simulink model "mpc_tgt_calc"  (R2022b)
settings: Solver=FixedStepDiscrete  StartTime=0.0  StopTime=2600  FixedStep=0.1  RelTol=1e-3
undefined symbols (not defined in the file): accl, alpha, alpha2, ang, beta, cnt_delay_accl_ratio, cnt_delay_decel_ratio, delay_accl, delay_v, dist, dt, ff_duty_l, ff_duty_r, ideal_point, img_ang, img_dist, kanayama_point, pivot_state, sla_param, slip, slip_point, state, trj_diff, v, vx, vy, w
(part 2 of 2)

== system mpc_tgt_calc/slalom/Subsystem2 ==
  ego : Inport
  tgt : Inport  Port=2
  Add : Sum
  Add1 : Sum
  Bus Selector : BusSelector  OutputSignals=w,sla_param,sla_param.counter
  Bus Selector1 : BusSelector  OutputSignals=sla_param.counter,sla_param.limit_time_count
  Constant1 : Constant  Value=0
  Data Store Read : DataStoreRead  DataStoreName=time_step  IndexOptions=Index vector (dialog)  Indices=1  OutputSizes=1
  Data Store Read1 : DataStoreRead  DataStoreName=time_step  IndexOptions=Index vector (dialog)  Indices=1  OutputSizes=1
  Data Type Conversion : DataTypeConversion  OutDataTypeStr=single  SaturateOnIntegerOverflow=off  RndMeth=Floor
  Data Type Conversion1 : DataTypeConversion  OutDataTypeStr=single  SaturateOnIntegerOverflow=off  RndMeth=Floor
  Data Type Conversion2 : DataTypeConversion  OutDataTypeStr=single  SaturateOnIntegerOverflow=off  RndMeth=Floor
  Gain : Gain  Gain=dt
  Product : Product
  Relational Operator : RelationalOperator  OutDataTypeStr=boolean  RndMeth=Simplest  InputSameDT=off
  Subsystem : Subsystem
  Switch : Switch  Criteria=u2 > Threshold  SaturateOnIntegerOverflow=off  InputSameDT=off
  Terminator : Terminator
  next_w : Outport
  next_alpha : Outport  Port=2
  next_count : Outport  Port=3
  next_alpha2 : Outport  Port=4
  wires:
  Bus Selector/1 -> Add/1  "<w>"
  Subsystem/1(next_alpha) -> next_alpha/1, Gain/1
  Bus Selector/2 -> Subsystem/1(ego)  "<sla_param>"
  Bus Selector/3 -> Add1/1  "<counter>"
  Data Store Read1/1 -> Data Type Conversion2/1
  Add1/1 -> Data Type Conversion1/1
  Data Type Conversion/1 -> Add/2
  Data Type Conversion2/1 -> Add1/2
  Data Type Conversion1/1 -> next_count/1
  tgt/1 -> Terminator/1
  Bus Selector1/2 -> Relational Operator/2  "<limit_time_count>"
  Relational Operator/1 -> Switch/2
  ego/1 -> Bus Selector1/1, Bus Selector/1
  Bus Selector1/1 -> Relational Operator/1  "<counter>"
  Constant1/1 -> Switch/1
  Add/1 -> Switch/3
  Switch/1 -> next_w/1
  Data Store Read/1 -> Product/1
  Gain/1 -> Product/2
  Product/1 -> Data Type Conversion/1
  Subsystem/2(next_alpha2) -> next_alpha2/1

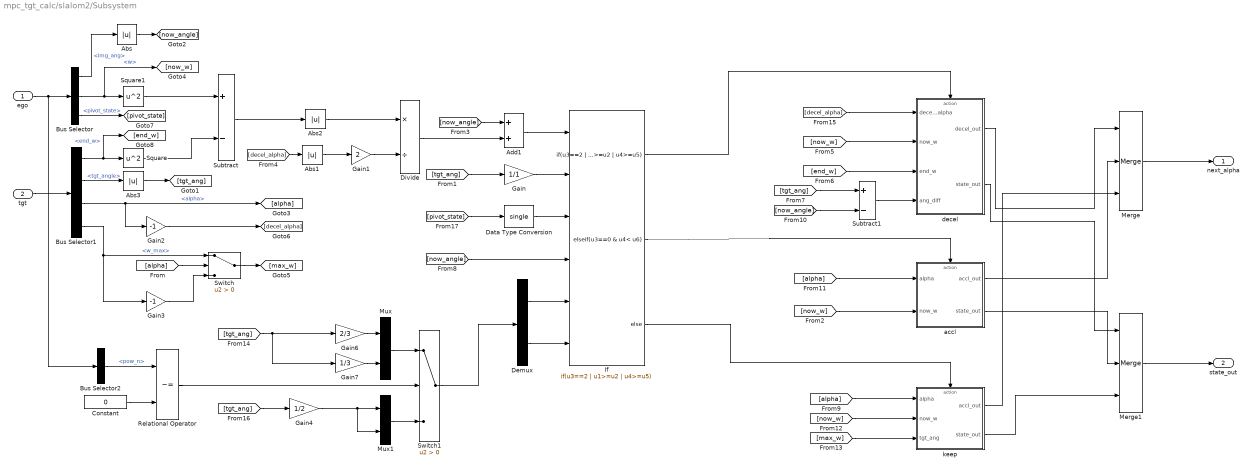
== system mpc_tgt_calc/slalom2/Subsystem ==
  ego : Inport
  tgt : Inport  Port=2
  Abs{,1..3} (4 alike) : Abs  SaturateOnIntegerOverflow=off
  Add1 : Sum
  Bus Selector : BusSelector  OutputSignals=img_ang,w,pivot_state
  Bus Selector1 : BusSelector  OutputSignals=end_w,tgt_angle,alpha,w_max
  Bus Selector2 : BusSelector  OutputSignals=sla_param.pow_n
  Constant : Constant  Value=0
  Data Type Conversion : DataTypeConversion  OutDataTypeStr=single  SaturateOnIntegerOverflow=off  RndMeth=Floor
  Demux : Demux  Outputs=2
  Divide : Product  Inputs=*/
  Gain : Gain  Gain=1/1
  Gain1 : Gain  Gain=2
  Gain2 : Gain  Gain=-1
  Gain3 : Gain  Gain=-1
  Gain4 : Gain  Gain=1/2
  Gain6 : Gain  Gain=2/3
  Gain7 : Gain  Gain=1/3
  If : If  NumInputs=6  IfExpression=u3==2 | u1>=u2 | u4>=u5  ElseIfExpressions=u3==0 & u4< u6
  Merge : Merge  Inputs=3
  Merge1 : Merge  Inputs=3
  Mux : Mux  Inputs=2
  Mux1 : Mux  Inputs=2
  Relational Operator : RelationalOperator  Operator=~=  OutDataTypeStr=boolean  RndMeth=Simplest  InputSameDT=off
  Square : Math  Operator=square
  Square1 : Math  Operator=square
  Subtract : Sum  Inputs=+-
  Subtract1 : Sum  Inputs=+-
  Switch : Switch  Criteria=u2 > Threshold  SaturateOnIntegerOverflow=off  InputSameDT=off
  Switch1 : Switch  Criteria=u2 > Threshold  SaturateOnIntegerOverflow=off  InputSameDT=off
  accl : Subsystem  TreatAsAtomicUnit=on
  decel : Subsystem  TreatAsAtomicUnit=on
  keep : Subsystem  TreatAsAtomicUnit=on
  next_alpha : Outport
  state_out : Outport  Port=2
  wires:
  ego/1 -> Bus Selector2/1, Bus Selector/1
  Subtract/1 -> Abs2/1
  Divide/1 -> Add1/2
  [now_angle] -> Add1/1
  Abs1/1 -> Gain1/1
  Abs2/1 -> Divide/1
  [decel_alpha] -> Abs1/1
  Gain1/1 -> Divide/2
  tgt/1 -> Bus Selector1/1
  Bus Selector1/1 -> [end_w], Square/1  "<end_w>"
  Square/1 -> Subtract/2
  Square1/1 -> Subtract/1
  Bus Selector/3 -> [pivot_state]  "<pivot_state>"
  Bus Selector/2 -> [now_w], Square1/1  "<w>"
  Bus Selector/1 -> Abs/1  "<img_ang>"
  Bus Selector1/2 -> Abs3/1  "<tgt_angle>"
  Bus Selector1/3 -> Gain2/1, [alpha]  "<alpha>"
  Gain2/1 -> [decel_alpha]
  Switch/1 -> [max_w]
  [alpha] -> Switch/2
  Bus Selector1/4 -> Gain3/1, Switch/1  "<w_max>"
  Gain3/1 -> Switch/3
  [pivot_state] -> Data Type Conversion/1
  Data Type Conversion/1 -> If/3
  Add1/1 -> If/1
  keep/2(state_out) -> Merge1/3
  decel/1(decel_out) -> Merge/1
  [max_w] -> keep/3(tgt_ang)
  accl/1(accl_out) -> Merge/2
  [now_w] -> keep/2(now_w)
  [decel_alpha] -> decel/1(decel_alpha)
  [now_w] -> decel/2(now_w)
  [now_angle] -> Subtract1/2
  [tgt_ang] -> Subtract1/1
  [now_w] -> accl/2(now_w)
  accl/2(state_out) -> Merge1/2
  If/2 -> accl/Action
  keep/1(accl_out) -> Merge/3
  [alpha] -> keep/1(alpha)
  If/3 -> keep/Action
  [end_w] -> decel/3(end_w)
  decel/2(state_out) -> Merge1/1
  Merge1/1 -> state_out/1
  Subtract1/1 -> decel/4(ang_diff)
  If/1 -> decel/Action
  Merge/1 -> next_alpha/1
  [alpha] -> accl/1(alpha)
  Abs/1 -> [now_angle]
  Abs3/1 -> [tgt_ang]
  Gain/1 -> If/2
  Demux/1 -> If/5
  [now_angle] -> If/4
  Demux/2 -> If/6
  [tgt_ang] -> Gain/1
  Gain7/1 -> Mux/2
  Gain6/1 -> Mux/1
  [tgt_ang] -> Gain6/1, Gain7/1
  Mux/1 -> Switch1/1
  Mux1/1 -> Switch1/3
  Gain4/1 -> Mux1/2, Mux1/1
  Switch1/1 -> Demux/1
  [tgt_ang] -> Gain4/1
  Bus Selector2/1 -> Relational Operator/1  "<pow_n>"
  Constant/1 -> Relational Operator/2
  Relational Operator/1 -> Switch1/2

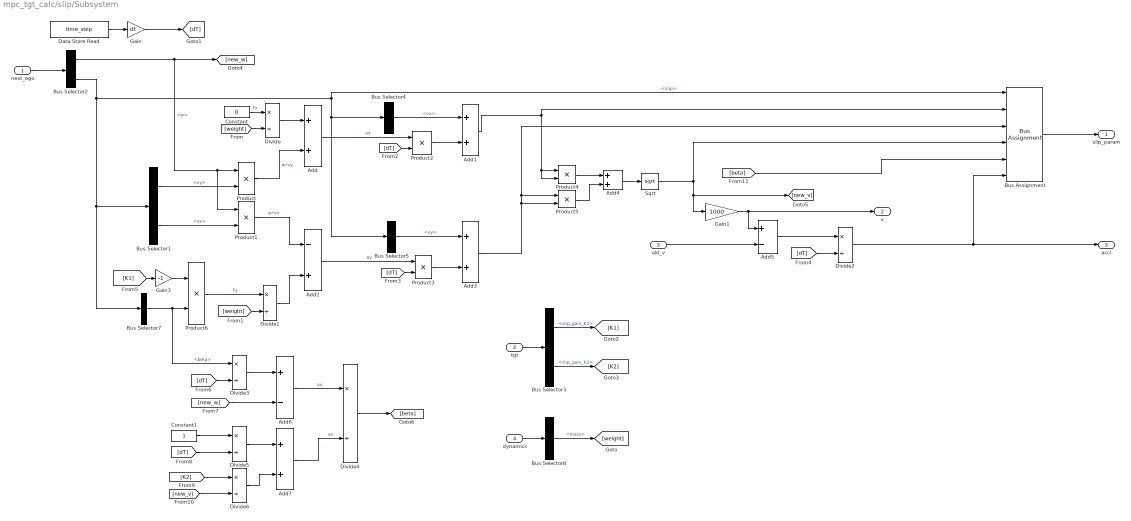
== system mpc_tgt_calc/slip/Subsystem ==
  next_ego : Inport
  tgt : Inport  Port=2
  old_v : Inport  Port=3
  dynamics : Inport  Port=4
  Add{,1,3..4,7} (5 alike) : Sum
  Add2 : Sum  Inputs=-+
  Add5 : Sum  Inputs=+-
  Add6 : Sum  Inputs=+-
  Bus Assignment : BusAssignment  AssignedSignals=vx,vy,v,beta,accl
  Bus Selector1 : BusSelector  OutputSignals=vy,vx
  Bus Selector2 : BusSelector  OutputSignals=w,slip
  Bus Selector3 : BusSelector  OutputSignals=slip_gain_K1,slip_gain_K2
  Bus Selector4 : BusSelector  OutputSignals=vx
  Bus Selector5 : BusSelector  OutputSignals=vy
  Bus Selector7 : BusSelector  OutputSignals=beta
  Bus Selector8 : BusSelector  OutputSignals=mass
  Constant : Constant  Value=0  OutDataTypeStr=single
  Constant1 : Constant  OutDataTypeStr=single
  Data Store Read : DataStoreRead  DataStoreName=time_step  IndexOptions=Index vector (dialog)  Indices=1  OutputSizes=1
  Divide{,1..6} (7 alike) : Product  Inputs=*/
  Gain : Gain  Gain=dt
  Gain1 : Gain  Gain=1000
  Gain3 : Gain  Gain=-1
  Product{,1..6} (7 alike) : Product
  Sqrt : Sqrt
  slip_param : Outport
  v : Outport  Port=2
  accl : Outport  Port=3
  wires:
  next_ego/1 -> Bus Selector2/1
  Bus Assignment/1 -> slip_param/1
  tgt/1 -> Bus Selector3/1
  Bus Selector2/1 -> [new_w], Product1/1, Product/1  "<w>"
  Bus Selector1/1 -> Product/2  "<vy>"
  Bus Selector1/2 -> Product1/2  "<vx>"
  Constant/1 -> Divide/1  "Fx"
  [weight] -> Divide/2
  [weight] -> Divide1/2
  Product/1 -> Add/2  "w*vy"
  Divide/1 -> Add/1
  Bus Selector4/1 -> Add1/1  "<vx>"
  Data Store Read/1 -> Gain/1
  Gain/1 -> [dT]
  Add/1 -> Product2/1  "ax"
  [dT] -> Product2/2
  Product2/1 -> Add1/2
  Add1/1 -> Product4/2, Product4/1, Bus Assignment/2
  Product3/1 -> Add3/2
  [dT] -> Product3/2
  Bus Selector2/2 -> Bus Selector7/1, Bus Selector1/1, Bus Assignment/1, Bus Selector4/1, Bus Selector5/1  "<slip>"
  Add3/1 -> Product5/1, Bus Assignment/3, Product5/2
  Add2/1 -> Product3/1  "ay"
  Bus Selector5/1 -> Add3/1  "<vy>"
  Product1/1 -> Add2/1  "w*vx"
  Product5/1 -> Add4/2
  Sqrt/1 -> [new_v], Gain1/1, Bus Assignment/4
  Add4/1 -> Sqrt/1
  Product4/1 -> Add4/1
  Gain1/1 -> Add5/1, v/1
  Divide1/1 -> Add2/2
  old_v/1 -> Add5/2
  Add5/1 -> Divide2/1
  [dT] -> Divide2/2
  Divide2/1 -> Bus Assignment/6, accl/1
  Bus Selector3/1 -> [K1]  "<slip_gain_K1>"
  Bus Selector3/2 -> [K2]  "<slip_gain_K2>"
  Gain3/1 -> Product6/1
  [K1] -> Gain3/1
  Bus Selector7/1 -> Divide3/1, Product6/2  "<beta>"
  Product6/1 -> Divide1/1  "Fy"
  [dT] -> Divide3/2
  [new_w] -> Add6/2
  Divide3/1 -> Add6/1
  Add6/1 -> Divide4/1  "ax"
  [dT] -> Divide5/2
  Constant1/1 -> Divide5/1
  Divide5/1 -> Add7/1
  Divide6/1 -> Add7/2
  Add7/1 -> Divide4/2  "ax"
  [K2] -> Divide6/1
  [new_v] -> Divide6/2
  Divide4/1 -> [beta]
  [beta] -> Bus Assignment/5
  dynamics/1 -> Bus Selector8/1
  Bus Selector8/1 -> [weight]  "<mass>"

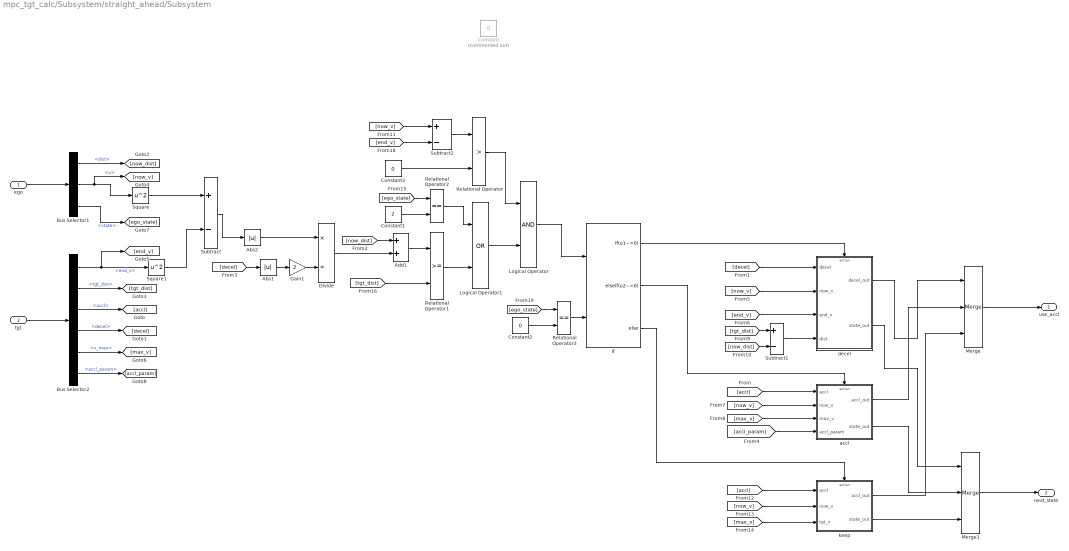
== system mpc_tgt_calc/Subsystem/straight_ahead/Subsystem ==
  ego : Inport
  tgt : Inport  Port=2
  Abs1 : Abs  SaturateOnIntegerOverflow=off
  Abs2 : Abs  SaturateOnIntegerOverflow=off
  Add1 : Sum
  Bus Selector1 : BusSelector  OutputSignals=dist,v,state
  Bus Selector2 : BusSelector  OutputSignals=end_v,tgt_dist,accl,decel,v_max,accl_param
  Constant : Constant  Commented=on  Value=0
  Constant1 : Constant  Value=2
  Constant2 : Constant  Value=0
  Constant3 : Constant  Value=0
  Divide : Product  Inputs=*/
  Gain1 : Gain  Gain=2
  If : If  NumInputs=2  IfExpression=u1~=0  ElseIfExpressions=u2~=0
  Logical Operator : Logic  AllPortsSameDT=off  OutDataTypeStr=boolean
  Logical Operator1 : Logic  Operator=OR  AllPortsSameDT=off  OutDataTypeStr=boolean
  Merge : Merge  Inputs=3
  Merge1 : Merge  Inputs=3
  Relational Operator : RelationalOperator  Operator=>  OutDataTypeStr=boolean  RndMeth=Simplest  InputSameDT=off
  Relational Operator1 : RelationalOperator  OutDataTypeStr=boolean  RndMeth=Simplest  InputSameDT=off
  Relational Operator2 : RelationalOperator  Operator===  OutDataTypeStr=boolean  RndMeth=Simplest  InputSameDT=off
  Relational Operator3 : RelationalOperator  Operator===  OutDataTypeStr=boolean  RndMeth=Simplest  InputSameDT=off
  Square : Math  Operator=square
  Square1 : Math  Operator=square
  Subtract : Sum  Inputs=+-
  Subtract1 : Sum  Inputs=+-
  Subtract2 : Sum  Inputs=+-
  accl : Subsystem  TreatAsAtomicUnit=on
  decel : Subsystem  TreatAsAtomicUnit=on
  keep : Subsystem  TreatAsAtomicUnit=on
  use_accl : Outport
  next_state : Outport  Port=2
  wires:
  Add1/1 -> Relational Operator1/1
  Gain1/1 -> Divide/2
  tgt/1 -> Bus Selector2/1
  [accl] -> accl/1(accl)
  [decel] -> decel/1(decel)
  Square/1 -> Subtract/1
  Divide/1 -> Add1/2
  Bus Selector2/1 -> [end_v], Square1/1  "<end_v>"
  ego/1 -> Bus Selector1/1
  Bus Selector1/2 -> Square/1, [now_v]  "<v>"
  Bus Selector2/3 -> [accl]  "<accl>"
  Bus Selector2/4 -> [decel]  "<decel>"
  Bus Selector1/1 -> [now_dist]  "<dist>"
  [now_dist] -> Add1/1
  [decel] -> Abs1/1
  Abs1/1 -> Gain1/1
  Subtract/1 -> Abs2/1
  Bus Selector2/2 -> [tgt_dist]  "<tgt_dist>"
  [now_v] -> decel/2(now_v)
  [end_v] -> decel/3(end_v)
  [now_v] -> accl/2(now_v)
  Bus Selector2/5 -> [max_v]  "<v_max>"
  Bus Selector1/3 -> [ego_state]  "<state>"
  Merge/1 -> use_accl/1
  [tgt_dist] -> Subtract1/1
  [now_dist] -> Subtract1/2
  Subtract1/1 -> decel/4(dist)
  [max_v] -> accl/3(max_v)
  If/3 -> keep/Action
  Merge1/1 -> next_state/1
  [accl] -> keep/1(accl)
  [now_v] -> keep/2(now_v)
  [max_v] -> keep/3(tgt_v)
  If/1 -> decel/Action
  If/2 -> accl/Action
  keep/1(accl_out) -> Merge/3
  decel/1(decel_out) -> Merge/1
  decel/2(state_out) -> Merge1/1
  keep/2(state_out) -> Merge1/3
  accl/1(accl_out) -> Merge/2
  accl/2(state_out) -> Merge1/2
  Bus Selector2/6 -> [accl_param]  "<accl_param>"
  [accl_param] -> accl/4(accl_param)
  [now_v] -> Subtract2/1
  [end_v] -> Subtract2/2
  Subtract2/1 -> Relational Operator/1
  Square1/1 -> Subtract/2
  Constant3/1 -> Relational Operator/2
  Relational Operator/1 -> Logical Operator/1
  [tgt_dist] -> Relational Operator1/2
  Relational Operator1/1 -> Logical Operator1/2
  [ego_state] -> Relational Operator2/1
  Constant1/1 -> Relational Operator2/2
  Relational Operator2/1 -> Logical Operator1/1
  Logical Operator1/1 -> Logical Operator/2
  Logical Operator/1 -> If/1
  [ego_state] -> Relational Operator3/1
  Relational Operator3/1 -> If/2
  Constant2/1 -> Relational Operator3/2
  Abs2/1 -> Divide/1

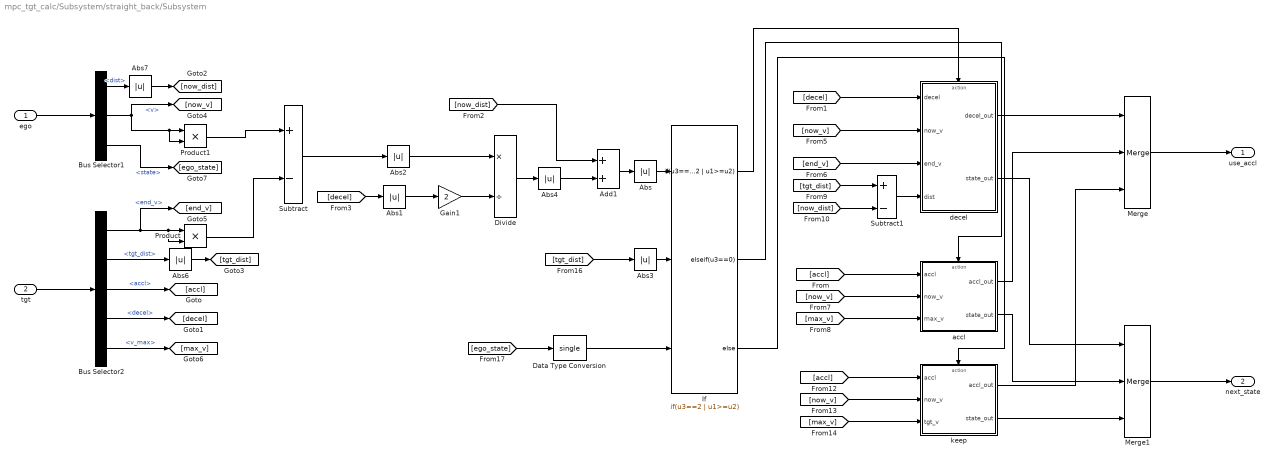
== system mpc_tgt_calc/Subsystem/straight_back/Subsystem ==
  ego : Inport
  tgt : Inport  Port=2
  Abs{,1..4,6..7} (7 alike) : Abs  SaturateOnIntegerOverflow=off
  Add1 : Sum
  Bus Selector1 : BusSelector  OutputSignals=dist,v,state
  Bus Selector2 : BusSelector  OutputSignals=end_v,tgt_dist,accl,decel,v_max
  Data Type Conversion : DataTypeConversion  OutDataTypeStr=single  SaturateOnIntegerOverflow=off  RndMeth=Floor
  Divide : Product  Inputs=*/
  Gain1 : Gain  Gain=2
  If : If  NumInputs=3  IfExpression=u3==2 | u1>=u2  ElseIfExpressions=u3==0
  Merge : Merge  Inputs=3
  Merge1 : Merge  Inputs=3
  Product : Product
  Product1 : Product
  Subtract : Sum  Inputs=+-
  Subtract1 : Sum  Inputs=+-
  accl : Subsystem  TreatAsAtomicUnit=on
  decel : Subsystem  TreatAsAtomicUnit=on
  keep : Subsystem  TreatAsAtomicUnit=on
  use_accl : Outport
  next_state : Outport  Port=2
  wires:
  Add1/1 -> Abs/1
  Gain1/1 -> Divide/2
  Product/1 -> Subtract/2
  Subtract/1 -> Abs2/1
  tgt/1 -> Bus Selector2/1
  [accl] -> accl/1(accl)
  [decel] -> decel/1(decel)
  Product1/1 -> Subtract/1
  Divide/1 -> Abs4/1
  Bus Selector2/1 -> Product/2, Product/1, [end_v]  "<end_v>"
  ego/1 -> Bus Selector1/1
  Bus Selector1/2 -> Product1/2, Product1/1, [now_v]  "<v>"
  Bus Selector2/3 -> [accl]  "<accl>"
  Bus Selector2/4 -> [decel]  "<decel>"
  Bus Selector1/1 -> Abs7/1  "<dist>"
  [decel] -> Abs1/1
  Abs1/1 -> Gain1/1
  Abs2/1 -> Divide/1
  Bus Selector2/2 -> Abs6/1  "<tgt_dist>"
  [now_v] -> decel/2(now_v)
  [end_v] -> decel/3(end_v)
  [now_v] -> accl/2(now_v)
  Bus Selector2/5 -> [max_v]  "<v_max>"
  Bus Selector1/3 -> [ego_state]  "<state>"
  Merge/1 -> use_accl/1
  [tgt_dist] -> Subtract1/1
  [now_dist] -> Subtract1/2
  Subtract1/1 -> decel/4(dist)
  [max_v] -> accl/3(max_v)
  If/3 -> keep/Action
  Merge1/1 -> next_state/1
  [accl] -> keep/1(accl)
  [now_v] -> keep/2(now_v)
  [max_v] -> keep/3(tgt_v)
  If/1 -> decel/Action
  If/2 -> accl/Action
  [tgt_dist] -> Abs3/1
  [ego_state] -> Data Type Conversion/1
  Data Type Conversion/1 -> If/3
  keep/1(accl_out) -> Merge/3
  decel/1(decel_out) -> Merge/1
  decel/2(state_out) -> Merge1/1
  keep/2(state_out) -> Merge1/3
  accl/1(accl_out) -> Merge/2
  accl/2(state_out) -> Merge1/2
  Abs/1 -> If/1
  Abs3/1 -> If/2
  Abs4/1 -> Add1/2
  [now_dist] -> Add1/1
  Abs6/1 -> [tgt_dist]
  Abs7/1 -> [now_dist]

== system mpc_tgt_calc/calc_FF/Subsystem/If Action Subsystem ==
  front_volt : Inport
  next_ego : Inport  Port=2
  Action Port : ActionPort  ActionPortLabel=if((u2==0 | u2==3 ) & (u1==0))
  Bus Selector : BusSelector  OutputSignals=ff_duty_low_v_th,ff_duty_low_th
  Bus Selector1 : BusSelector  OutputSignals=v
  Max : MinMax  Function=max  Inputs=2
  Mux : Mux  Inputs=2
  Relational Operator : RelationalOperator  Operator=>  OutDataTypeStr=boolean  RndMeth=Simplest  InputSameDT=off
  Scope : Scope  NumInputPorts=4
  Switch : Switch  Criteria=u2 > Threshold  SaturateOnIntegerOverflow=off  InputSameDT=off
  Out1 : Outport
  wires:
  next_ego/1 -> Bus Selector/1, Bus Selector1/1
  Bus Selector1/1 -> Mux/1, Relational Operator/1  "<v>"
  Bus Selector/1 -> Mux/2, Relational Operator/2  "<ff_duty_low_v_th>"
  Relational Operator/1 -> Scope/3, Switch/2
  front_volt/1 -> Max/1, Switch/1
  Bus Selector/2 -> Max/2  "<ff_duty_low_th>"
  Switch/1 -> Scope/1, Out1/1
  Max/1 -> Scope/2, Switch/3
  Mux/1 -> Scope/4

== system mpc_tgt_calc/calc_FF/Subsystem/If Action Subsystem1 ==
  front_volt : Inport
  Action Port : ActionPort  ActionPortLabel=else
  Out1 : Outport
  wires:
  front_volt/1 -> Out1/1

== system mpc_tgt_calc/pivot/Subsystem/accl ==
  alpha : Inport
  now_w : Inport  Port=2
  max_w : Inport  Port=3
  Action Port : ActionPort  ActionPortLabel=elseif(u3==0 )
  Abs : Abs  SaturateOnIntegerOverflow=off
  Abs1 : Abs  SaturateOnIntegerOverflow=off
  Constant : Constant  Value=0
  Constant1 : Constant  Value=0  OutDataTypeStr=int32
  Constant2 : Constant  OutDataTypeStr=int32
  Constant3 : Constant  OutDataTypeStr=single
  Constant4 : Constant  Value=2.5  OutDataTypeStr=single
  Data Type Conversion : DataTypeConversion  OutDataTypeStr=single  SaturateOnIntegerOverflow=off  RndMeth=Floor
  Divide : Product  Inputs=*/
  Manual Switch : ManualSwitch
  Product1 : Product
  Relational Operator : RelationalOperator  Operator=<  OutDataTypeStr=boolean  RndMeth=Simplest  InputSameDT=off
  Square : Math  Operator=pow
  Subtract : Sum  Inputs=+-
  Switch : Switch  Criteria=u2 > Threshold  SaturateOnIntegerOverflow=off  InputSameDT=off
  Switch1 : Switch  Criteria=u2 > Threshold  SaturateOnIntegerOverflow=off  InputSameDT=off
  accl_out : Outport
  state_out : Outport  Port=2
  wires:
  Switch/1 -> Data Type Conversion/1
  Relational Operator/1 -> Switch1/2, Switch/2
  max_w/1 -> Divide/2, Abs1/1
  Constant/1 -> Switch/3
  alpha/1 -> [alpha], Manual Switch/1, Product1/1
  Constant1/1 -> Switch1/1
  Constant2/1 -> Switch1/3
  Constant3/1 -> Subtract/1
  Divide/1 -> Square/1
  Square/1 -> Subtract/2
  Subtract/1 -> Product1/2
  Constant4/1 -> Square/2
  Product1/1 -> Manual Switch/2
  Manual Switch/1 -> Switch/1
  now_w/1 -> Abs/1, Divide/1
  Switch1/1 -> state_out/1
  Data Type Conversion/1 -> accl_out/1
  Abs/1 -> Relational Operator/1
  Abs1/1 -> Relational Operator/2

== system mpc_tgt_calc/pivot/Subsystem/decel ==
  decel_alpha : Inport
  now_w : Inport  Port=2
  end_w : Inport  Port=3
  ang : Inport  Port=4
  Action Port : ActionPort  ActionPortLabel=if(u3==2 | u1>=u2)
  Abs : Abs  SaturateOnIntegerOverflow=off
  Abs1 : Abs  SaturateOnIntegerOverflow=off
  Abs2 : Abs  SaturateOnIntegerOverflow=off
  Constant : Constant  Value=0  OutDataTypeStr=single
  Constant1 : Constant  Value=0.01*2*pi/360
  Constant2 : Constant  Value=2  OutDataTypeStr=int32
  Data Type Conversion : DataTypeConversion  OutDataTypeStr=single  SaturateOnIntegerOverflow=off  RndMeth=Floor
  Divide : Product  Inputs=*/
  Gain : Gain  Gain=2
  Gain1 : Gain  Gain=-1
  Manual Switch : ManualSwitch  CurrentSetting=0
  Min : MinMax  Function=max  Inputs=2
  Relational Operator : RelationalOperator  Operator=>  OutDataTypeStr=boolean  RndMeth=Simplest  InputSameDT=off
  Relational Operator1 : RelationalOperator  Operator=<  OutDataTypeStr=boolean  RndMeth=Simplest  InputSameDT=off
  Relational Operator2 : RelationalOperator  Operator=<  OutDataTypeStr=boolean  RndMeth=Simplest  InputSameDT=off
  Square : Math  Operator=square
  Square1 : Math  Operator=square
  Subtract : Sum  Inputs=+-
  Switch{,1..3} (4 alike) : Switch  Criteria=u2 > Threshold  SaturateOnIntegerOverflow=off  InputSameDT=off
  decel_out : Outport
  state_out : Outport  Port=2
  wires:
  Square1/1 -> Subtract/2
  Constant1/1 -> Min/1
  Min/1 -> Gain/1
  Subtract/1 -> Divide/1
  Constant/1 -> Switch/3
  Gain/1 -> Divide/2
  Divide/1 -> Abs/1
  ang/1 -> Min/2
  Square/1 -> Subtract/1
  Constant2/1 -> state_out/1
  end_w/1 -> Relational Operator/2, Relational Operator1/2, Square1/1
  now_w/1 -> Relational Operator/1, Relational Operator1/1, Square/1
  [decel_alpha] -> Switch2/2
  Relational Operator/1 -> Switch2/3
  Relational Operator1/1 -> Switch2/1
  Switch1/1 -> Manual Switch/2
  Abs/1 -> Data Type Conversion/1
  Gain1/1 -> Switch1/3
  Switch2/1 -> Switch/2
  Switch/1 -> decel_out/1
  Data Type Conversion/1 -> Gain1/1, Switch1/1
  Manual Switch/1 -> Switch/1, Abs1/1
  decel_alpha/1 -> [decel_alpha], Switch1/2, Switch3/1, Abs2/1, Manual Switch/1
  Abs2/1 -> Relational Operator2/1
  Relational Operator2/1 -> Switch3/2
  Abs1/1 -> Relational Operator2/2

== system mpc_tgt_calc/pivot/Subsystem/keep ==
  alpha : Inport
  now_w : Inport  Port=2
  tgt_ang : Inport  Port=3
  Action Port : ActionPort  ActionPortLabel=else
  Constant : Constant  Value=0
  Constant2 : Constant  OutDataTypeStr=int32
  Data Type Conversion : DataTypeConversion  OutDataTypeStr=single  SaturateOnIntegerOverflow=off  RndMeth=Floor
  Terminator : Terminator
  Terminator1 : Terminator
  Terminator2 : Terminator
  accl_out : Outport
  state_out : Outport  Port=2
  wires:
  Constant2/1 -> state_out/1
  Constant/1 -> Data Type Conversion/1
  Data Type Conversion/1 -> accl_out/1
  alpha/1 -> Terminator/1
  now_w/1 -> Terminator1/1
  tgt_ang/1 -> Terminator2/1

== system mpc_tgt_calc/slalom/Subsystem2/Subsystem ==
  ego : Inport
  Add : Sum
  Add1 : Sum
  Bus Selector : BusSelector  OutputSignals=state,base_alpha,counter,limit_time_count
  Constant : Constant  Value=0  OutDataTypeStr=single
  Data Store Read1 : DataStoreRead  DataStoreName=time_step  IndexOptions=Index vector (dialog)  Indices=1  OutputSizes=1
  Data Store Read2 : DataStoreRead  DataStoreName=time_step2  IndexOptions=Index vector (dialog)  Indices=1  OutputSizes=1
  If : If  IfExpression=u1 ~= 0
  If Action Subsystem : Subsystem  TreatAsAtomicUnit=on
  If Action Subsystem1 : Subsystem  TreatAsAtomicUnit=on
  If Action Subsystem2 : Subsystem  TreatAsAtomicUnit=on
  If Action Subsystem3 : Subsystem  TreatAsAtomicUnit=on
  If2 : If  IfExpression=u1 ~= 0
  Merge : Merge
  Merge1 : Merge
  Product : Product
  Product1 : Product
  Relational Operator : RelationalOperator  Operator=>  OutDataTypeStr=boolean  RndMeth=Simplest  InputSameDT=off
  Relational Operator1 : RelationalOperator  Operator=>  OutDataTypeStr=boolean  RndMeth=Simplest  InputSameDT=off
  Switch : Switch  Criteria=u2 ~= 0  SaturateOnIntegerOverflow=off  InputSameDT=off
  Switch3 : Switch  Criteria=u2 ~= 0  SaturateOnIntegerOverflow=off  InputSameDT=off
  next_alpha : Outport
  next_alpha2 : Outport  Port=2
  wires:
  ego/1 -> If Action Subsystem3/1(ego), If Action Subsystem1/1(ego), Bus Selector/1
  Bus Selector/1 -> Switch3/2, Switch/2  "<state>"
  Switch/1 -> next_alpha/1
  Constant/1 -> Switch3/1, Switch/1
  Bus Selector/2 -> Product1/1, Product/1  "<base_alpha>"
  Product/1 -> Switch/3
  Merge/1 -> Product/2
  Relational Operator/1 -> If/1
  Bus Selector/4 -> Relational Operator1/2, Relational Operator/2  "<limit_time_count>"
  Data Store Read1/1 -> Add/1
  Bus Selector/3 -> Add1/2, Add/2  "<counter>"
  Add/1 -> Relational Operator/1
  Product1/1 -> Switch3/3
  Switch3/1 -> next_alpha2/1
  Data Store Read2/1 -> Add1/1
  Add1/1 -> Relational Operator1/1
  If/1 -> If Action Subsystem/Action
  Relational Operator1/1 -> If2/1
  If/2 -> If Action Subsystem1/Action
  If Action Subsystem/1(Out1) -> Merge/1
  If Action Subsystem1/1(neipier) -> Merge/2
  If Action Subsystem2/1(Out1) -> Merge1/1
  If2/1 -> If Action Subsystem2/Action
  If Action Subsystem3/1(neipier) -> Merge1/2
  If2/2 -> If Action Subsystem3/Action
  Merge1/1 -> Product1/2

== system mpc_tgt_calc/slalom2/Subsystem/accl ==
  alpha : Inport
  now_w : Inport  Port=2
  Action Port : ActionPort  ActionPortLabel=elseif(u3==0 & u4< u6)
  Constant1 : Constant  Value=0  OutDataTypeStr=int32
  Data Type Conversion : DataTypeConversion  OutDataTypeStr=single  SaturateOnIntegerOverflow=off  RndMeth=Floor
  Terminator : Terminator
  accl_out : Outport
  state_out : Outport  Port=2
  wires:
  alpha/1 -> Data Type Conversion/1
  Constant1/1 -> state_out/1
  Data Type Conversion/1 -> accl_out/1
  now_w/1 -> Terminator/1

== system mpc_tgt_calc/slalom2/Subsystem/decel ==
  decel_alpha : Inport
  now_w : Inport  Port=2
  end_w : Inport  Port=3
  ang_diff : Inport  Port=4
  Action Port : ActionPort  ActionPortLabel=if(u3==2 | u1>=u2 | u4>=u5)
  Abs : Abs  SaturateOnIntegerOverflow=off
  Constant : Constant  Value=0  OutDataTypeStr=single
  Constant1 : Constant  Value=0.1*pi/180
  Constant2 : Constant  Value=2  OutDataTypeStr=int32
  Constant3 : Constant  Commented=on  Value=0.75
  Data Type Conversion : DataTypeConversion  OutDataTypeStr=single  SaturateOnIntegerOverflow=off  RndMeth=Floor
  Divide : Product  Inputs=*/
  From1 : From  Commented=on  GotoTag=ang_diff_abs
  Gain : Gain  Gain=2
  Gain1 : Gain  Gain=-1
  Min : MinMax  Function=max  Inputs=2
  Relational Operator : RelationalOperator  Operator=>  OutDataTypeStr=boolean  RndMeth=Simplest  InputSameDT=off
  Relational Operator1 : RelationalOperator  Operator=<  OutDataTypeStr=boolean  RndMeth=Simplest  InputSameDT=off
  Relational Operator2 : RelationalOperator  Commented=on  Operator=>  OutDataTypeStr=boolean  RndMeth=Simplest  InputSameDT=off
  Square : Math  Operator=square
  Square1 : Math  Operator=square
  Subtract : Sum  Inputs=+-
  Switch : Switch  Criteria=u2 > Threshold  SaturateOnIntegerOverflow=off  InputSameDT=off
  Switch1 : Switch  Criteria=u2 > Threshold  SaturateOnIntegerOverflow=off  InputSameDT=off
  Switch2 : Switch  Criteria=u2 > Threshold  SaturateOnIntegerOverflow=off  InputSameDT=off
  Switch3 : Switch  Commented=on  Criteria=u2 > Threshold  SaturateOnIntegerOverflow=off  InputSameDT=off
  decel_out : Outport
  state_out : Outport  Port=2
  wires:
  Square1/1 -> Subtract/2
  ang_diff/1 -> Min/1
  Min/1 -> Gain/1
  Subtract/1 -> Divide/1
  Constant/1 -> Switch/3
  Gain/1 -> Divide/2
  Divide/1 -> Abs/1
  Square/1 -> Subtract/1
  Constant2/1 -> state_out/1
  decel_alpha/1 -> [decel_alpha], Switch1/2, Switch3/1
  end_w/1 -> Relational Operator/2, Relational Operator1/2, Square1/1
  now_w/1 -> Relational Operator/1, Relational Operator1/1, Square/1
  [decel_alpha] -> Switch2/2
  Relational Operator/1 -> Switch2/3
  Relational Operator1/1 -> Switch2/1
  Switch1/1 -> Switch/1
  Abs/1 -> Data Type Conversion/1
  Gain1/1 -> Switch1/3
  Switch2/1 -> Switch/2
  Switch/1 -> decel_out/1
  Data Type Conversion/1 -> Gain1/1, Switch1/1
  From1/1 -> Relational Operator2/1
  Constant3/1 -> Relational Operator2/2
  Relational Operator2/1 -> Switch3/2
  Constant1/1 -> Min/2

== system mpc_tgt_calc/slalom2/Subsystem/keep ==
  alpha : Inport
  now_w : Inport  Port=2
  tgt_ang : Inport  Port=3
  Action Port : ActionPort  ActionPortLabel=else
  Constant : Constant  Value=0
  Constant2 : Constant  OutDataTypeStr=int32
  Data Type Conversion : DataTypeConversion  OutDataTypeStr=single  SaturateOnIntegerOverflow=off  RndMeth=Floor
  Terminator : Terminator
  Terminator1 : Terminator
  Terminator2 : Terminator
  accl_out : Outport
  state_out : Outport  Port=2
  wires:
  Constant2/1 -> state_out/1
  Constant/1 -> Data Type Conversion/1
  Data Type Conversion/1 -> accl_out/1
  alpha/1 -> Terminator/1
  now_w/1 -> Terminator1/1
  tgt_ang/1 -> Terminator2/1

== system mpc_tgt_calc/Subsystem/straight_ahead/Subsystem/accl ==
  accl : Inport
  now_v : Inport  Port=2
  max_v : Inport  Port=3
  accl_param : Inport  Port=4
  Action Port : ActionPort  ActionPortLabel=elseif(u2~=0 )
  Bus Selector : BusSelector  OutputSignals=limit,n
  Constant : Constant  Value=0
  Constant1 : Constant  Value=0  OutDataTypeStr=int32
  Constant2 : Constant  OutDataTypeStr=int32
  Constant3 : Constant  OutDataTypeStr=single
  Data Type Conversion : DataTypeConversion  OutDataTypeStr=single  SaturateOnIntegerOverflow=off  RndMeth=Floor
  Divide : Product  Inputs=*/
  Product1 : Product
  Relational Operator : RelationalOperator  Operator=<  OutDataTypeStr=boolean  RndMeth=Simplest  InputSameDT=off
  Relational Operator1 : RelationalOperator  Operator=>  OutDataTypeStr=boolean  RndMeth=Simplest  InputSameDT=off
  Square : Math  Operator=pow
  Subtract : Sum  Inputs=+-
  Switch : Switch  Criteria=u2 > Threshold  SaturateOnIntegerOverflow=off  InputSameDT=off
  Switch1 : Switch  Criteria=u2 > Threshold  SaturateOnIntegerOverflow=off  InputSameDT=off
  Switch2 : Switch  Criteria=u2 > Threshold  SaturateOnIntegerOverflow=off  InputSameDT=off
  accl_out : Outport
  state_out : Outport  Port=2
  wires:
  Switch/1 -> Data Type Conversion/1
  now_v/1 -> Relational Operator1/1, Relational Operator/1, Divide/1
  Relational Operator/1 -> Switch/2, Switch1/2
  max_v/1 -> Relational Operator/2, Divide/2
  Constant/1 -> Switch/3
  Data Type Conversion/1 -> accl_out/1
  accl/1 -> Switch2/3, Product1/1
  Switch1/1 -> state_out/1
  Constant1/1 -> Switch1/1
  Constant2/1 -> Switch1/3
  Constant3/1 -> Subtract/1
  Divide/1 -> Square/1
  Square/1 -> Subtract/2
  Subtract/1 -> Product1/2
  [n] -> Square/2
  Switch2/1 -> Switch/1
  Product1/1 -> Switch2/1
  Relational Operator1/1 -> Switch2/2
  accl_param/1 -> Bus Selector/1
  Bus Selector/1 -> [limit]  "<limit>"
  Bus Selector/2 -> [n]  "<n>"
  [limit] -> Relational Operator1/2

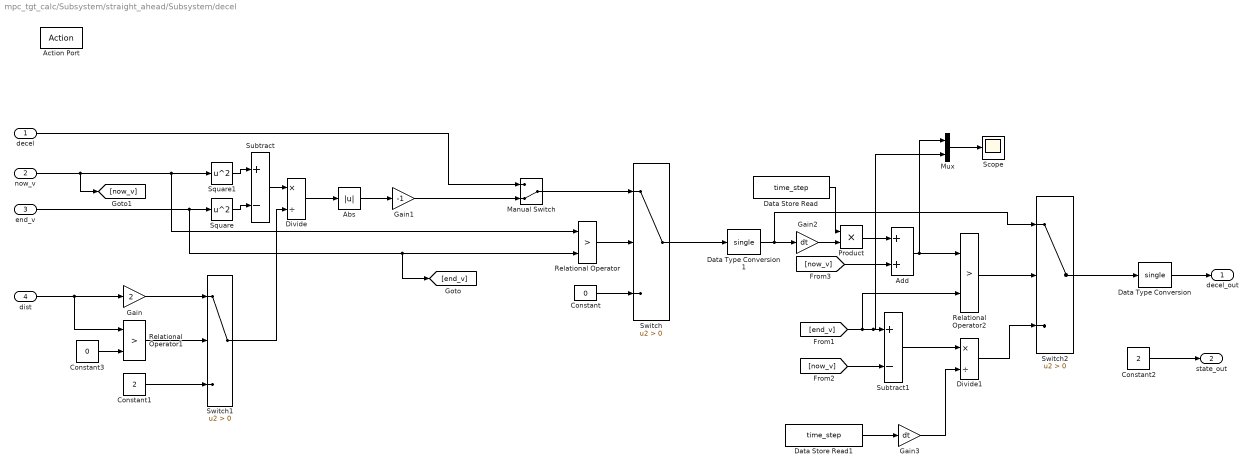
== system mpc_tgt_calc/Subsystem/straight_ahead/Subsystem/decel ==
  decel : Inport
  now_v : Inport  Port=2
  end_v : Inport  Port=3
  dist : Inport  Port=4
  Action Port : ActionPort  ActionPortLabel=if(u1~=0)
  Abs : Abs  SaturateOnIntegerOverflow=off
  Add : Sum
  Constant : Constant  Value=0
  Constant1 : Constant  Value=2
  Constant2 : Constant  Value=2  OutDataTypeStr=int32
  Constant3 : Constant  Value=0
  Data Store Read : DataStoreRead  DataStoreName=time_step  IndexOptions=Index vector (dialog)  Indices=1  OutputSizes=1
  Data Store Read1 : DataStoreRead  DataStoreName=time_step  IndexOptions=Index vector (dialog)  Indices=1  OutputSizes=1
  Data Type Conversion : DataTypeConversion  OutDataTypeStr=single  SaturateOnIntegerOverflow=off  RndMeth=Floor
  Data Type Conversion1 : DataTypeConversion  OutDataTypeStr=single  SaturateOnIntegerOverflow=off  RndMeth=Floor
  Divide : Product  Inputs=*/
  Divide1 : Product  Inputs=*/
  Gain : Gain  Gain=2
  Gain1 : Gain  Gain=-1
  Gain2 : Gain  Gain=dt
  Gain3 : Gain  Gain=dt
  Manual Switch : ManualSwitch  CurrentSetting=0
  Mux : Mux  Inputs=2
  Product : Product
  Relational Operator : RelationalOperator  Operator=>  OutDataTypeStr=boolean  RndMeth=Simplest  InputSameDT=off
  Relational Operator1 : RelationalOperator  Operator=>  OutDataTypeStr=boolean  RndMeth=Simplest  InputSameDT=off
  Relational Operator2 : RelationalOperator  Operator=>  OutDataTypeStr=boolean  RndMeth=Simplest  InputSameDT=off
  Scope : Scope
  Square : Math  Operator=square
  Square1 : Math  Operator=square
  Subtract : Sum  Inputs=+-
  Subtract1 : Sum  Inputs=+-
  Switch : Switch  Criteria=u2 > Threshold  SaturateOnIntegerOverflow=off  InputSameDT=off
  Switch1 : Switch  Criteria=u2 > Threshold  SaturateOnIntegerOverflow=off  InputSameDT=off
  Switch2 : Switch  Criteria=u2 > Threshold  SaturateOnIntegerOverflow=off  InputSameDT=off
  decel_out : Outport
  state_out : Outport  Port=2
  wires:
  Square/1 -> Subtract/2
  dist/1 -> Gain/1, Relational Operator1/1
  Abs/1 -> Gain1/1
  Gain1/1 -> Manual Switch/2
  Relational Operator/1 -> Switch/2
  Subtract/1 -> Divide/1
  Constant/1 -> Switch/3
  Gain/1 -> Switch1/1
  Divide/1 -> Abs/1
  Square1/1 -> Subtract/1
  Constant2/1 -> state_out/1
  Manual Switch/1 -> Switch/1
  decel/1 -> Manual Switch/1
  end_v/1 -> Square/1, [end_v], Relational Operator/2
  Constant3/1 -> Relational Operator1/2
  Relational Operator1/1 -> Switch1/2
  Switch1/1 -> Divide/2
  Constant1/1 -> Switch1/3
  now_v/1 -> [now_v], Square1/1, Relational Operator/1
  Gain2/1 -> Product/2
  Data Store Read/1 -> Product/1
  Data Type Conversion1/1 -> Switch2/1, Gain2/1
  Product/1 -> Add/1
  [now_v] -> Add/2
  Add/1 -> Mux/1, Relational Operator2/1
  Relational Operator2/1 -> Switch2/2
  Data Type Conversion/1 -> decel_out/1
  Switch2/1 -> Data Type Conversion/1
  [end_v] -> Relational Operator2/2, Mux/2, Subtract1/1
  [now_v] -> Subtract1/2
  Gain3/1 -> Divide1/2
  Subtract1/1 -> Divide1/1
  Data Store Read1/1 -> Gain3/1
  Divide1/1 -> Switch2/3
  Mux/1 -> Scope/1
  Switch/1 -> Data Type Conversion1/1

== system mpc_tgt_calc/Subsystem/straight_ahead/Subsystem/keep ==
  accl : Inport
  now_v : Inport  Port=2
  tgt_v : Inport  Port=3
  Action Port : ActionPort  ActionPortLabel=else
  Constant : Constant  Value=0
  Constant2 : Constant  OutDataTypeStr=int32
  Data Type Conversion : DataTypeConversion  OutDataTypeStr=single  SaturateOnIntegerOverflow=off  RndMeth=Floor
  Terminator : Terminator
  Terminator1 : Terminator
  Terminator2 : Terminator
  accl_out : Outport
  state_out : Outport  Port=2
  wires:
  Constant2/1 -> state_out/1
  Constant/1 -> Data Type Conversion/1
  Data Type Conversion/1 -> accl_out/1
  accl/1 -> Terminator/1
  now_v/1 -> Terminator1/1
  tgt_v/1 -> Terminator2/1

== system mpc_tgt_calc/Subsystem/straight_back/Subsystem/accl ==
  accl : Inport
  now_v : Inport  Port=2
  max_v : Inport  Port=3
  Action Port : ActionPort  ActionPortLabel=elseif(u3==0 )
  Constant : Constant  Value=0
  Constant1 : Constant  Value=0  OutDataTypeStr=int32
  Constant2 : Constant  OutDataTypeStr=int32
  Constant3 : Constant  OutDataTypeStr=single
  Constant4 : Constant  Value=2.5  OutDataTypeStr=single
  Data Type Conversion : DataTypeConversion  OutDataTypeStr=single  SaturateOnIntegerOverflow=off  RndMeth=Floor
  Divide : Product  Inputs=*/
  Manual Switch : ManualSwitch  CurrentSetting=0
  Product1 : Product
  Relational Operator : RelationalOperator  Operator=>  OutDataTypeStr=boolean  RndMeth=Simplest  InputSameDT=off
  Square : Math  Operator=pow
  Subtract : Sum  Inputs=+-
  Switch : Switch  Criteria=u2 > Threshold  SaturateOnIntegerOverflow=off  InputSameDT=off
  Switch1 : Switch  Criteria=u2 > Threshold  SaturateOnIntegerOverflow=off  InputSameDT=off
  accl_out : Outport
  state_out : Outport  Port=2
  wires:
  Switch/1 -> Data Type Conversion/1
  now_v/1 -> Relational Operator/1, Divide/1
  Relational Operator/1 -> Switch/2, Switch1/2
  max_v/1 -> Relational Operator/2, Divide/2
  Constant/1 -> Switch/3
  Data Type Conversion/1 -> accl_out/1
  accl/1 -> Manual Switch/1, Product1/1
  Switch1/1 -> state_out/1
  Constant1/1 -> Switch1/1
  Constant2/1 -> Switch1/3
  Constant3/1 -> Subtract/1
  Divide/1 -> Square/1
  Square/1 -> Subtract/2
  Subtract/1 -> Product1/2
  Constant4/1 -> Square/2
  Manual Switch/1 -> Switch/1
  Product1/1 -> Manual Switch/2

== system mpc_tgt_calc/Subsystem/straight_back/Subsystem/decel ==
  decel : Inport
  now_v : Inport  Port=2
  end_v : Inport  Port=3
  dist : Inport  Port=4
  Action Port : ActionPort  ActionPortLabel=if(u3==2 | u1>=u2)
  Abs : Abs  SaturateOnIntegerOverflow=off
  Constant : Constant  Value=0
  Constant1 : Constant  Value=0.01
  Constant2 : Constant  Value=2  OutDataTypeStr=int32
  Data Type Conversion : DataTypeConversion  OutDataTypeStr=single  SaturateOnIntegerOverflow=off  RndMeth=Floor
  Divide : Product  Inputs=*/
  Gain : Gain  Gain=2
  Gain1 : Gain
  Manual Switch : ManualSwitch  CurrentSetting=0
  Min : MinMax  Function=max  Inputs=2
  Relational Operator : RelationalOperator  Operator=<  OutDataTypeStr=boolean  RndMeth=Simplest  InputSameDT=off
  Square : Math  Operator=square
  Square1 : Math  Operator=square
  Subtract : Sum  Inputs=+-
  Switch : Switch  Criteria=u2 > Threshold  SaturateOnIntegerOverflow=off  InputSameDT=off
  decel_out : Outport
  state_out : Outport  Port=2
  wires:
  Square1/1 -> Subtract/2
  Constant1/1 -> Min/1
  Abs/1 -> Gain1/1
  Gain1/1 -> Manual Switch/2
  Min/1 -> Gain/1
  Switch/1 -> Data Type Conversion/1
  Relational Operator/1 -> Switch/2
  Subtract/1 -> Divide/1
  Constant/1 -> Switch/3
  Gain/1 -> Divide/2
  Divide/1 -> Abs/1
  dist/1 -> Min/2
  Square/1 -> Subtract/1
  Constant2/1 -> state_out/1
  Data Type Conversion/1 -> decel_out/1
  Manual Switch/1 -> Switch/1
  decel/1 -> Manual Switch/1
  end_v/1 -> Relational Operator/2, Square1/1
  now_v/1 -> Relational Operator/1, Square/1

== system mpc_tgt_calc/Subsystem/straight_back/Subsystem/keep ==
  accl : Inport
  now_v : Inport  Port=2
  tgt_v : Inport  Port=3
  Action Port : ActionPort  ActionPortLabel=else
  Constant : Constant  Value=0
  Constant2 : Constant  OutDataTypeStr=int32
  Data Type Conversion : DataTypeConversion  OutDataTypeStr=single  SaturateOnIntegerOverflow=off  RndMeth=Floor
  Terminator : Terminator
  Terminator1 : Terminator
  Terminator2 : Terminator
  accl_out : Outport
  state_out : Outport  Port=2
  wires:
  Constant2/1 -> state_out/1
  Constant/1 -> Data Type Conversion/1
  Data Type Conversion/1 -> accl_out/1
  accl/1 -> Terminator/1
  now_v/1 -> Terminator1/1
  tgt_v/1 -> Terminator2/1

== system mpc_tgt_calc/slalom/Subsystem2/Subsystem/If Action Subsystem ==
  Action Port : ActionPort  ActionPortLabel=if(u1 ~= 0)
  Constant1 : Constant  Value=0  OutDataTypeStr=single
  Out1 : Outport
  wires:
  Constant1/1 -> Out1/1

== system mpc_tgt_calc/slalom/Subsystem2/Subsystem/If Action Subsystem1 ==
  ego : Inport
  Action Port : ActionPort  ActionPortLabel=else
  calc_neiper : Subsystem
  neipier : Outport
  wires:
  ego/1 -> calc_neiper/1(ego)
  calc_neiper/1(neipier) -> neipier/1

== system mpc_tgt_calc/slalom/Subsystem2/Subsystem/If Action Subsystem2 ==
  Action Port : ActionPort  ActionPortLabel=if(u1 ~= 0)
  Constant1 : Constant  Value=0  OutDataTypeStr=single
  Out1 : Outport
  wires:
  Constant1/1 -> Out1/1

== system mpc_tgt_calc/slalom/Subsystem2/Subsystem/If Action Subsystem3 ==
  ego : Inport
  Action Port : ActionPort  ActionPortLabel=else
  calc_neiper1 : Subsystem
  neipier : Outport
  wires:
  ego/1 -> calc_neiper1/1(ego)
  calc_neiper1/1(neipier) -> neipier/1

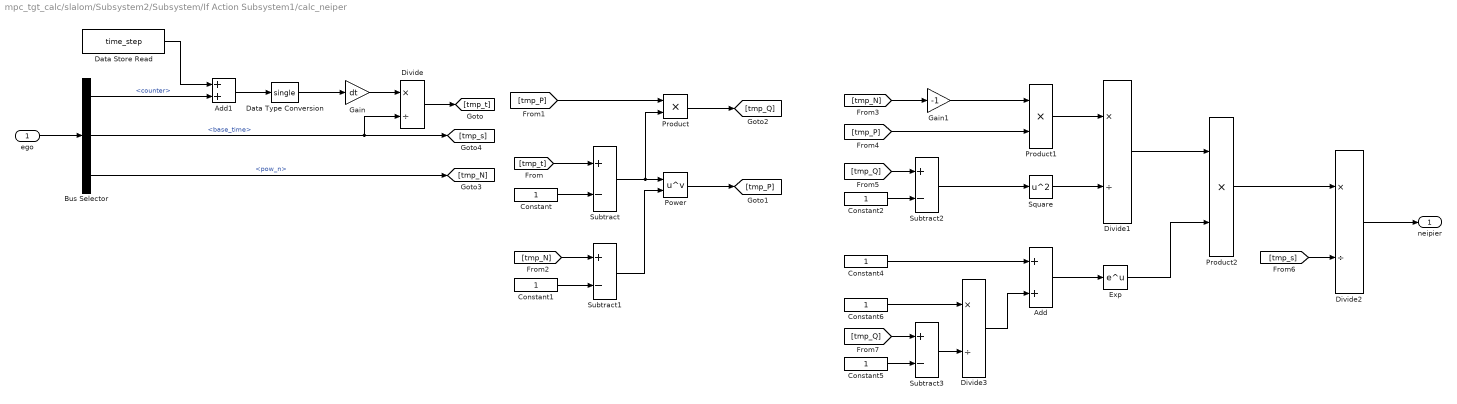
== system mpc_tgt_calc/slalom/Subsystem2/Subsystem/If Action Subsystem1/calc_neiper ==
  ego : Inport
  Add : Sum
  Add1 : Sum
  Bus Selector : BusSelector  OutputSignals=counter,base_time,pow_n
  Constant{,1..2,4..6} (6 alike) : Constant  OutDataTypeStr=single
  Data Store Read : DataStoreRead  DataStoreName=time_step  IndexOptions=Index vector (dialog)  Indices=1  OutputSizes=1
  Data Type Conversion : DataTypeConversion  OutDataTypeStr=single  SaturateOnIntegerOverflow=off  RndMeth=Floor
  Divide{,1..3} (4 alike) : Product  Inputs=*/
  Exp : Math
  Gain : Gain  Gain=dt
  Gain1 : Gain  Gain=-1
  Power : Math  Operator=pow
  Product : Product
  Product1 : Product
  Product2 : Product
  Square : Math  Operator=square
  Subtract{,1..3} (4 alike) : Sum  Inputs=+-
  neipier : Outport
  wires:
  ego/1 -> Bus Selector/1
  Gain/1 -> Divide/1
  Bus Selector/2 -> Divide/2, [tmp_s]  "<base_time>"
  Divide/1 -> [tmp_t]
  [tmp_t] -> Subtract/1
  Constant/1 -> Subtract/2
  Subtract/1 -> Power/1, Product/2
  Subtract1/1 -> Power/2
  Constant1/1 -> Subtract1/2
  Power/1 -> [tmp_P]
  [tmp_P] -> Product/1
  Product/1 -> [tmp_Q]
  Bus Selector/3 -> [tmp_N]  "<pow_n>"
  [tmp_N] -> Subtract1/1
  [tmp_N] -> Gain1/1
  Gain1/1 -> Product1/1
  [tmp_P] -> Product1/2
  Product1/1 -> Divide1/1
  [tmp_Q] -> Subtract2/1
  Constant2/1 -> Subtract2/2
  Subtract2/1 -> Square/1
  Square/1 -> Divide1/2
  Divide1/1 -> Product2/1
  Product2/1 -> Divide2/1
  [tmp_s] -> Divide2/2
  Constant4/1 -> Add/1
  [tmp_Q] -> Subtract3/1
  Constant5/1 -> Subtract3/2
  Divide3/1 -> Add/2
  Subtract3/1 -> Divide3/2
  Constant6/1 -> Divide3/1
  Add/1 -> Exp/1
  Exp/1 -> Product2/2
  Divide2/1 -> neipier/1
  Bus Selector/1 -> Add1/2  "<counter>"
  Data Type Conversion/1 -> Gain/1
  Data Store Read/1 -> Add1/1
  Add1/1 -> Data Type Conversion/1

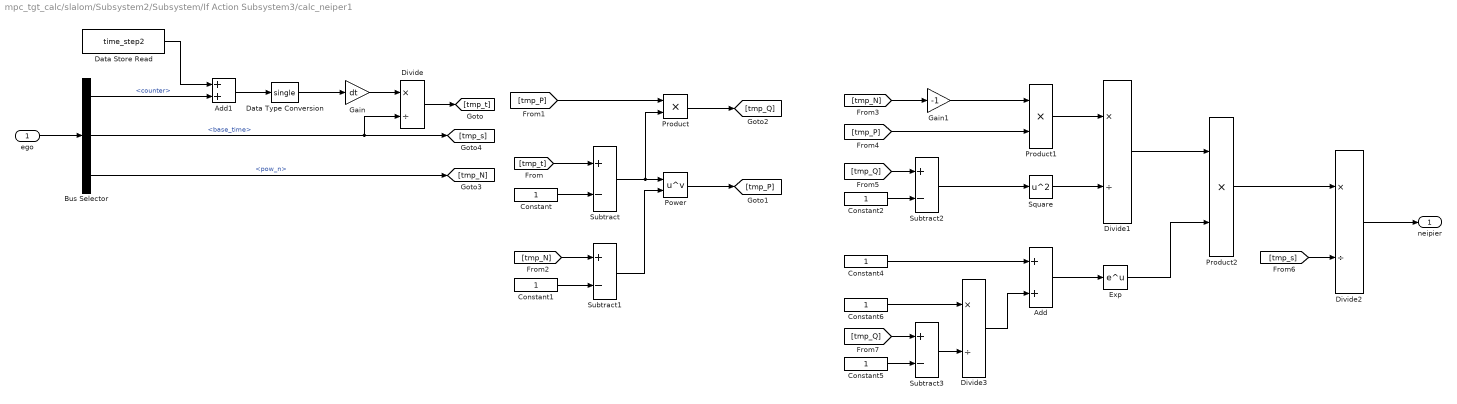
== system mpc_tgt_calc/slalom/Subsystem2/Subsystem/If Action Subsystem3/calc_neiper1 ==
  ego : Inport
  Add : Sum
  Add1 : Sum
  Bus Selector : BusSelector  OutputSignals=counter,base_time,pow_n
  Constant{,1..2,4..6} (6 alike) : Constant  OutDataTypeStr=single
  Data Store Read : DataStoreRead  DataStoreName=time_step2  IndexOptions=Index vector (dialog)  Indices=1  OutputSizes=1
  Data Type Conversion : DataTypeConversion  OutDataTypeStr=single  SaturateOnIntegerOverflow=off  RndMeth=Floor
  Divide{,1..3} (4 alike) : Product  Inputs=*/
  Exp : Math
  Gain : Gain  Gain=dt
  Gain1 : Gain  Gain=-1
  Power : Math  Operator=pow
  Product : Product
  Product1 : Product
  Product2 : Product
  Square : Math  Operator=square
  Subtract{,1..3} (4 alike) : Sum  Inputs=+-
  neipier : Outport
  wires:
  ego/1 -> Bus Selector/1
  Gain/1 -> Divide/1
  Bus Selector/2 -> Divide/2, [tmp_s]  "<base_time>"
  Divide/1 -> [tmp_t]
  [tmp_t] -> Subtract/1
  Constant/1 -> Subtract/2
  Subtract/1 -> Power/1, Product/2
  Subtract1/1 -> Power/2
  Constant1/1 -> Subtract1/2
  Power/1 -> [tmp_P]
  [tmp_P] -> Product/1
  Product/1 -> [tmp_Q]
  Bus Selector/3 -> [tmp_N]  "<pow_n>"
  [tmp_N] -> Subtract1/1
  [tmp_N] -> Gain1/1
  Gain1/1 -> Product1/1
  [tmp_P] -> Product1/2
  Product1/1 -> Divide1/1
  [tmp_Q] -> Subtract2/1
  Constant2/1 -> Subtract2/2
  Subtract2/1 -> Square/1
  Square/1 -> Divide1/2
  Divide1/1 -> Product2/1
  Product2/1 -> Divide2/1
  [tmp_s] -> Divide2/2
  Constant4/1 -> Add/1
  [tmp_Q] -> Subtract3/1
  Constant5/1 -> Subtract3/2
  Divide3/1 -> Add/2
  Subtract3/1 -> Divide3/2
  Constant6/1 -> Divide3/1
  Add/1 -> Exp/1
  Exp/1 -> Product2/2
  Divide2/1 -> neipier/1
  Bus Selector/1 -> Add1/2  "<counter>"
  Data Type Conversion/1 -> Gain/1
  Data Store Read/1 -> Add1/1
  Add1/1 -> Data Type Conversion/1

== matlab function mpc_tgt_calc/kanayama_ctrl_method1/MATLAB Function ==
  data: x output; ego input Bus: t_ego; y output; theta output; tgt input Bus: t_tgt
function [x, y,theta]  = detect_trj_point_impl(ego, tgt)
    [x, y, ~, theta, ~] = detect_trj_point(ego, tgt);
end
